simulink model "induction"  (R2021a)
settings: Solver=VariableStepAuto  StartTime=0.0  StopTime=15  RelTol=1e-3
libraries: spsACVoltageSourceLib x3, spsAsynchronousMachinepuUnitsLib x1, spsGroundLib x1, spspowerguiLib x1
settings Model: SimulationMode=accelerator  Creator=Abdullah123  LastModifiedBy=Abdullah123

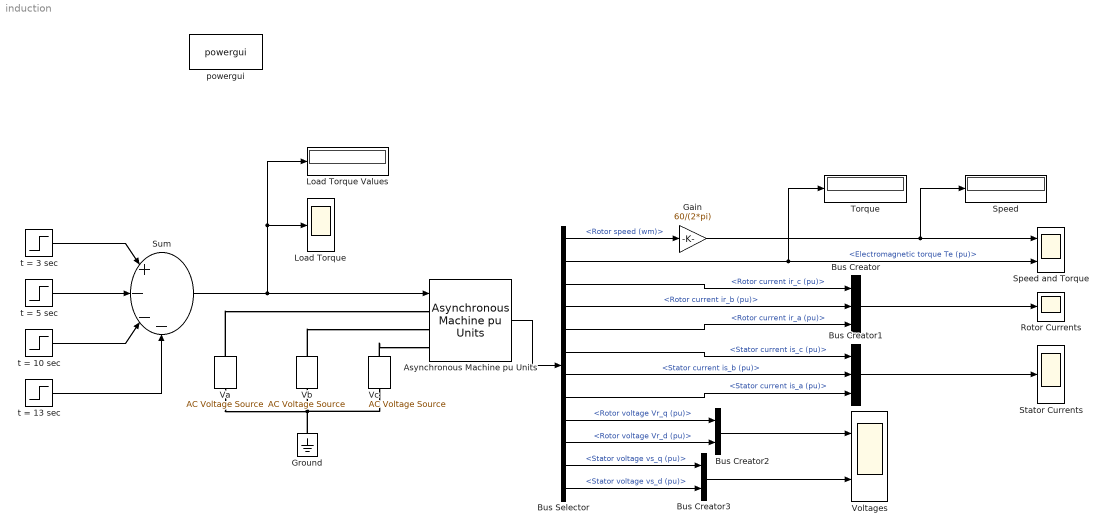
== system induction ==
  Asynchronous Machine pu Units : spsAsynchronousMachinepuUnitsLib/Asynchronous Machine pu Units  RotorType=Squirrel-cage  PresetModel="15:  5.4 HP (4KW)   400 V  50Hz 1430 RPM"  MechanicalLoad=Torque Tm  ShowDetailedParameters=on  ReferenceFrame=Rotor  Units=pu  MeasurementBus=off  NominalParameters=[4000 400 50]  VoltageRatio=1  Stator=[0.03513 0.04586]  Rotor=[0.03488 0.04586]  Cage1=[0.01909 0.0397]  Cage2=[0.01909 0.0397]  Lm=1.352  Mechanical=[0.0404 0.01841 2]  PolePairs=2  InitialConditions="[ 1,0   0,0,0   0,0,0 ]"  SimulateSaturation=off  Saturation="[0.212,0.4201,0.8125,1.0979,1.4799,2.2457,3.2586,4.5763,6.4763 ;   0.5,0.7,0.9,1,1.1,1.2 ,1.3,1.4,1.5]"  LoadFlowParameters=0  TsPowergui=0  TsBlock=-1  IterativeModel=Trapezoidal non iterative  IterativeDiscreteModel=Trapezoidal non iterative  Pmec=0
      settings: SourceProductBaseCode=PS
  Bus Creator : BusCreator  Inputs=3
  Bus Creator1 : BusCreator  Inputs=3
  Bus Creator2 : BusCreator  Inputs=2
  Bus Creator3 : BusCreator  Inputs=2
  Bus Selector : BusSelector  OutputSignals=Mechanical.Rotor speed (wm),Mechanical.Electromagnetic torque Te (pu),Rotor measurements.Rotor current ir_c (pu),Rotor measurements.Rotor current ir_b (pu),Rotor measurements.Rotor current ir_a (pu),Stator measurements.Stator current is_c (pu),Stator measurements.Stator current is_b (pu),Stator measurements.Stator current is_a (pu),Rotor measurements.Rotor voltage Vr_q (pu),Rotor measurements.Rotor voltage Vr_d (pu),Stator measurements.Stator voltage vs_q (pu),Stator measurements.Stator voltage vs_d (pu)
  Gain : Gain  Gain=60/(2*pi)
  Ground : spsGroundLib/Ground  LConnTagsString=a
  Load Torque : Scope
  Load Torque Values : Display
  Rotor Currents : Scope
  Speed : Display
  Speed and Torque : Scope  NumInputPorts=2
  Stator Currents : Scope
  Sum : Sum  Inputs=|+---
  Torque : Display
  Va : spsACVoltageSourceLib/AC Voltage Source  Amplitude=380  Phase=0  Frequency=50  SampleTime=0  Measurements=None  BusType=swing  Pref=10e3  Qref=0  Qmin=-inf  Qmax=+inf
  Vb : spsACVoltageSourceLib/AC Voltage Source  Amplitude=380  Phase=-120  Frequency=50  SampleTime=0  Measurements=None  BusType=swing  Pref=10e3  Qref=0  Qmin=-inf  Qmax=+inf
  Vc : spsACVoltageSourceLib/AC Voltage Source  Amplitude=380  Phase=120  Frequency=50  SampleTime=0  Measurements=None  BusType=swing  Pref=10e3  Qref=0  Qmin=-inf  Qmax=+inf
  Voltages : Scope  NumInputPorts=2
  powergui : spspowerguiLib/powergui  Priority=1  SimulationMode=Continuous  SampleTime=50e-6  frequency=60  Iterations=50  frequencyindice=50  Pbase=100e6  ErrMax=1e-4  UnitsV=kV  UnitsW=MW  buscounter=0  FunctionMessages=off  echomessages=off  EnableUseOfTLC=off  CurrentSourceSwitches=off  DisableSnubberDevices=off  DisableRonSwitches=off  DisableVfSwitches=off  DisplayEquations=off  AutomaticDiscreteSolvers=off  SolverType=Tustin/Backward Euler (TBE)  Interpol=off  ExternalGateDelay=off  methode=off  Ts=100  x0status=blocks  SPID=on  SwTol=0  HookPort=off  NonlinearTolerance=1e-4  nMaxIteration=100  ContinueOnMaxIteration=off  RestoreLinks=warning  ResistiveCurrentMeasurement=off  Frange=[0:2:500]  Ylog=off  Xlog=on  ShowGrid=off  save=off  variable=ZData  structure=0  ZoomFFT=off  StartTime=0.0  cycles=1  DisplayStyle=1  fundamental=60  FreqAxis=off  MaxFrequency=1000  frequencyindicesteady=1  RmsSteady=1  display=off
  t = 10 sec : Step  Time=10  After=6.68  SampleTime=0
  t = 13 sec : Step  Time=13  After=6.68  SampleTime=0
  t = 3 sec : Step  Time=3  After=26.72  SampleTime=0
  t = 5 sec : Step  Time=5  After=13.36  SampleTime=0
  wires:
  Asynchronous Machine pu Units/1 -> Bus Selector/1
  Bus Selector/1 -> Gain/1  "<Rotor speed (wm)>"
  Bus Selector/2 -> Torque/1, Speed and Torque/2  "<Electromagnetic torque Te (pu)>"
  Bus Selector/3 -> Bus Creator/1  "<Rotor current ir_c (pu)>"
  Bus Selector/4 -> Bus Creator/2  "<Rotor current ir_b (pu)>"
  Bus Selector/5 -> Bus Creator/3  "<Rotor current ir_a (pu)>"
  Bus Selector/8 -> Bus Creator1/3  "<Stator current is_a (pu)>"
  Bus Selector/7 -> Bus Creator1/2  "<Stator current is_b (pu)>"
  Bus Selector/6 -> Bus Creator1/1  "<Stator current is_c (pu)>"
  Bus Creator1/1 -> Stator Currents/1
  Gain/1 -> Speed/1, Speed and Torque/1
  Sum/1 -> Asynchronous Machine pu Units/1, Load Torque Values/1, Load Torque/1
  t = 5 sec/1 -> Sum/2
  t = 3 sec/1 -> Sum/1
  t = 10 sec/1 -> Sum/3
  t = 13 sec/1 -> Sum/4
  Bus Selector/9 -> Bus Creator2/1  "<Rotor voltage Vr_q (pu)>"
  Bus Selector/10 -> Bus Creator2/2  "<Rotor voltage Vr_d (pu)>"
  Bus Selector/12 -> Bus Creator3/2  "<Stator voltage vs_d (pu)>"
  Bus Selector/11 -> Bus Creator3/1  "<Stator voltage vs_q (pu)>"
  Bus Creator2/1 -> Voltages/1
  Bus Creator3/1 -> Voltages/2
  Bus Creator/1 -> Rotor Currents/1
  connections:
  Va/RConn1 -- Asynchronous Machine pu Units/LConn1
  Vb/RConn1 -- Asynchronous Machine pu Units/LConn2
  Vc/RConn1 -- Asynchronous Machine pu Units/LConn3
  Ground/LConn1 -- Va/LConn1 -- Vc/LConn1 -- Vb/LConn1
